simulink model "pll_d1"  (Simulink 7.4)
settings: Solver=ode45  StartTime=0.0  StopTime=6e-4  MaxStep=1/(10*50e6)  RelTol=1e-5  AbsTol=1e-6
PreLoadFcn:
  | load f_inv;   % 1/f filter kernel
undefined symbols (not defined in the file or in its folder): dfilt, One, sided
libraries: powerlib x11, dsparch4 x5, dspstat3 x5, simulink x4, simulink_extras x2, dspsnks4 x2, dspsrcs4 x1, dspbuff3 x1
settings Model: Creator=dbenson  LastModifiedBy=Dick  ExtModeTrigMode=oneshot  ExtModeArmWhenConnect=off
settings DataIOCC: LimitDataPoints=off  SaveOutput=off  SaveTime=off  SignalLoggingName=sigsOut
settings OptimizationCC: BooleanDataType=off  InitFltsAndDblsToZero=on
settings DebuggingCC: SaveWithParameterizedLinksMsg=none  SignalResolutionControl=TryResolveAllWithWarning  SolverPrmCheckMsg=none  MultiTaskDSMMsg=warning  MultiTaskCondExecSysMsg=none  StrictBusMsg=None
settings HardwareCC: TargetUnknown=on
settings RTWCC: RTWVerbose=off  IncludeERTFirstTime=on
settings CodeAppCC: GenerateComments=off  SimulinkBlockComments=off
settings GRTTargetCC: TargetFcnLib=ansi_tfl_tmw.mat

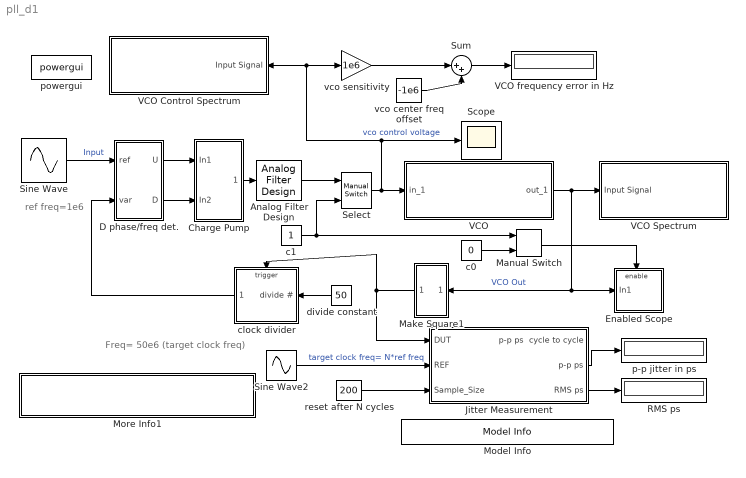
== system pll_d1 ==
  note: ref freq=1e6
  note: Freq= 50e6 (target clock freq)
  Analog Filter Design : dsparch4/Analog Filter Design  method=Butterworth  filttype=Lowpass  N=3  Wlo=2*pi*500e3  Whi=80  Rp=2  Rs=40
  Charge Pump : Subsystem  mask(RC Charge Pump){V=5}
      mask prompts: V "Output Voltage, V (Volts)"
  "D phase/freq det. " : Subsystem
  Enabled Scope : Subsystem  TreatAsAtomicUnit=on
  "Jitter Measurement " : Subsystem
  Make Square1 : Subsystem
      mask Type: Make Square
      mask Description:
      | For input +ve values output is 1
      | For input -ve values output is 0
      mask Display: plot(0,0,100,100,[90,70,70,50,50,30,30,10,10],[20,20,40,40,20,20,40,40,20],[90,87,84,80,76,73,70,67,63,60,57,53,50,47,44,40,36,33,30,27,23,20,17,13,10],[70,65,63,62,63,65,70,75,77,78,77,75,70,65,63,62,63,65,70,75,77,78,77,75,70])
  Manual Switch : simulink/Signal Routing/Manual Switch  SystemSampleTime=-1  sw=0  action=0  varsize=off
  Model Info : simulink/Model-Wide Utilities/Model Info  SystemSampleTime=-1  InitialBlockCM=none  BlockCM=none  Frame=on  DisplayStringWithTags=Copywrite 2005-2010 The MathWorks, Inc.  HorizontalTextAlignment=Center  LeftAlignmentValue=0.5  SourceBlockDiagram=pll_d1  TagMaxNumber=20
  More Info1 : Subsystem  AncestorBlock=rab_favorites/More Info1
      mask Display: disp(' x50  PLL model \n with time and \nfrequency domain measurements. ')
  RMS ps : Display
  Scope : Scope
      settings: TimeRange=0.0006  YMin=0  YMax=1.4  MaxDataPoints=50000  Decimation=500
  "Select " : simulink/Signal Routing/Manual Switch  SystemSampleTime=-1  sw=1  action=0  varsize=off
  Sine Wave : Sin  Amplitude=1  Bias=0  Frequency=2*pi*(1e6)  Phase=0  Samples=10  SampleTime=0  Offset=0
  Sine Wave2 : Sin  Amplitude=1  Bias=0  Frequency=2*pi*(50e6)  Phase=pi/2  Samples=10  SampleTime=0  Offset=0
  Sum : Sum  Inputs=|++  OutDataType=sfix(16)  OutScaling=2^0  SaturateOnIntegerOverflow=on  InputSameDT=on  OutDataTypeStr=Inherit: Same as first input
  VCO : Subsystem  mask{BW=100e3, Nrms=0 % 0.5, Ph=0, Kc=1e6, Fc=49e6, Ac=1}
      mask prompts: BW "Single Sided Noise BW (Hz)"; Nrms "Phase Noise Level (rms rad)"; Ph "Initial Phase (rad)"; Kc "Input Sensitivity (Hz/Volt)"; Fc "Oscillation freq (Hz)"; Ac "Output amplitude (Volt)"
      mask init:
      | pi2=2*pi;
      mask Display: disp('VCO with \n 1/F phase noise')
  VCO Control Spectrum : Subsystem  Description=Spectrum Analyzer  mask{BW=5e6}
      mask prompts: BW "Bandwidth"
      mask Display: fprintf('Baseband Spectrum Analyzer \n  BW=%7.2f MHz', BW/1e6)
  VCO Spectrum : Subsystem  Description=Spectrum Analyzer  mask{BW=5e6, Fc=1e6*50}
      mask prompts: BW "Bandwidth"; Fc "Center Freq"
      mask Display: fprintf('Spectrum Analyzer \n Fc=%7.2f MHz \n BW=%7.2f MHz',Fc/1e6,BW/1e6)
  VCO frequency error in Hz : Display
      settings: Decimation=401
  c0 : Constant  Value=0  OutDataType=sfix(16)  OutScaling=2^0
  c1 : Constant  OutDataType=sfix(16)  OutScaling=2^0
  clock divider : Subsystem  TreatAsAtomicUnit=on
  divide constant : Constant  Value=50  OutDataType=sfix(16)  OutScaling=2^0
  p-p jitter in ps : Display
  powergui : powerlib/powergui  SystemSampleTime=-1  SimulationMode=Continuous  SampleTime=0  frequency=60  SPID=off  DisableSnubberDevices=off  DisableRonSwitches=off  DisableVfSwitches=off  SwTol=0  Interpol=off  frequencyindice=0  echomessages=off  HookPort=off  DisplayEquations=off  FunctionMessages=off  EnableUseOfTLC=off  x0status=blocks  RestoreLinks=warning  Frange=[0:2:500]  Ylog=off  Xlog=on  ShowGrid=off  save=off  variable=ZData  ZoomFFT=on  StartTime=0.0  cycles=1  DisplayStyle=1  fundamental=60  FreqAxis=off  MaxFrequency=1000  frequencyindicesteady=1  RmsSteady=1  display=off  Ts=0  methode=off
  reset after N cycles : Constant  Value=200  VectorParams1D=off  OutDataType=sfix(16)  OutScaling=2^0
  vco center freq offset : Constant  Value=-1e6  OutDataType=sfix(16)  OutScaling=2^0
  vco sensitivity : Gain  Gain=1e6  ParameterDataType=sfix(16)  ParameterScaling=2^0  OutDataType=sfix(16)  OutScaling=2^0  SaturateOnIntegerOverflow=on  OutDataTypeStr=Inherit: Same as input  ParamDataTypeStr=Inherit: Same as input
  wires:
  Make Square1/1(Out1) -> clock divider/Trigger, "Jitter Measurement "/1(DUT)
  clock divider/1(" ") -> "D phase/freq det. "/2(var)
  Sine Wave/1 -> "D phase/freq det. "/1(ref)  "Input"
  Charge Pump/1(Out1) -> Analog Filter Design/1
  vco center freq offset/1 -> Sum/2
  Sum/1 -> VCO frequency error in Hz/1
  vco sensitivity/1 -> Sum/1
  VCO/1(out_1) -> VCO Spectrum/1(Input Signal), Make Square1/1(In1), Enabled Scope/1(In1)  "VCO Out"
  "Select "/1 -> Scope/1, vco sensitivity/1, VCO Control Spectrum/1(Input Signal), VCO/1(in_1)  "vco control voltage"
  c1/1 -> "Select "/2, Manual Switch/1
  "D phase/freq det. "/1(U) -> Charge Pump/1(In1)
  "D phase/freq det. "/2(D) -> Charge Pump/2(In2)
  Analog Filter Design/1 -> "Select "/1
  divide constant/1 -> clock divider/1("divide # ")
  Sine Wave2/1 -> "Jitter Measurement "/2(REF)  "target clock freq= N*ref freq"
  reset after N cycles/1 -> "Jitter Measurement "/3(Sample_Size)
  "Jitter Measurement "/2(p-p ps) -> p-p jitter in ps/1
  Manual Switch/1 -> Enabled Scope/Enable
  c0/1 -> Manual Switch/2
  "Jitter Measurement "/3(RMS ps) -> RMS ps/1

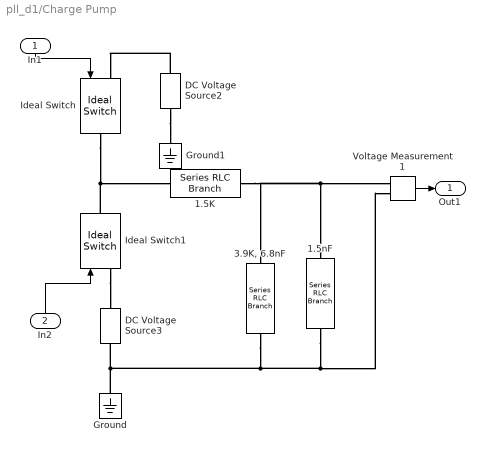
== system pll_d1/Charge Pump ==
  In1 : Inport  OutDataType=sfix(16)  OutScaling=2^0
  In2 : Inport  Port=2  OutDataType=sfix(16)  OutScaling=2^0
  1.5K : powerlib/Elements/Series RLC Branch  DialogController=POWERSYS.PowerSysDialog  PhysicalDomain=powersysdomain  SubClassName=unknown  LeftPortType=p1  RightPortType=p1  LConnTagsString=__new0  RConnTagsString=__new0  BranchType=R  Resistance=1500  Inductance=1e-3  SetiL0=off  InitialCurrent=0  Capacitance=1e-6  Setx0=off  InitialVoltage=0  Measurements=None
  1.5nF : powerlib/Elements/Series RLC Branch  DialogController=POWERSYS.PowerSysDialog  PhysicalDomain=powersysdomain  SubClassName=unknown  LeftPortType=p1  RightPortType=p1  LConnTagsString=__new0  RConnTagsString=__new0  BranchType=C  Resistance=3900  Inductance=1e-3  SetiL0=off  InitialCurrent=0  Capacitance=1.5e-9  Setx0=off  InitialVoltage=0  Measurements=None
  "3.9K, 6.8nF" : powerlib/Elements/Series RLC Branch  DialogController=POWERSYS.PowerSysDialog  PhysicalDomain=powersysdomain  SubClassName=unknown  LeftPortType=p1  RightPortType=p1  LConnTagsString=__new0  RConnTagsString=__new0  BranchType=RC  Resistance=3900  Inductance=1e-3  SetiL0=off  InitialCurrent=0  Capacitance=6.8e-9  Setx0=off  InitialVoltage=0  Measurements=None
  DC Voltage Source2 : powerlib/Electrical Sources/DC Voltage Source  DialogController=POWERSYS.PowerSysDialog  SystemSampleTime=-1  Amplitude=V  Measurements=None
  DC Voltage Source3 : powerlib/Electrical Sources/DC Voltage Source  DialogController=POWERSYS.PowerSysDialog  SystemSampleTime=-1  Amplitude=-V  Measurements=None
  Ground : powerlib/Elements/Ground  DialogController=POWERSYS.PowerSysDialog  PhysicalDomain=powersysdomain  SubClassName=unknown  LeftPortType=p1  RightPortType=p1  LConnTagsString=a
  Ground1 : powerlib/Elements/Ground  DialogController=POWERSYS.PowerSysDialog  PhysicalDomain=powersysdomain  SubClassName=unknown  LeftPortType=p1  RightPortType=p1  LConnTagsString=a
  Ideal Switch : powerlib/Power Electronics/Ideal Switch  DialogController=POWERSYS.PowerSysDialog  SystemSampleTime=-1  Ron=10  Lon=0  IC=0  Rs=inf  Cs=inf  Measurements=off
  Ideal Switch1 : powerlib/Power Electronics/Ideal Switch  DialogController=POWERSYS.PowerSysDialog  SystemSampleTime=-1  Ron=10  Lon=0  IC=0  Rs=inf  Cs=inf  Measurements=off
  Voltage Measurement1 : powerlib/Measurements/Voltage Measurement  DialogController=POWERSYS.PowerSysDialog  SystemSampleTime=-1  PhasorSimulation=off  OutputType=Complex  PSBequivalent=0
  Out1 : Outport  OutDataType=sfix(16)  OutScaling=2^0
  wires:
  In2/1 -> Ideal Switch1/1
  Voltage Measurement1/1 -> Out1/1
  In1/1 -> Ideal Switch/1
  connections:
  1.5nF/RConn1 -- "3.9K, 6.8nF"/RConn1 -- Ground/LConn1 -- DC Voltage Source3/LConn1 -- Voltage Measurement1/LConn2
  1.5K/RConn1 -- "3.9K, 6.8nF"/LConn1 -- Voltage Measurement1/LConn1 -- 1.5nF/LConn1
  Ideal Switch/RConn1 -- 1.5K/LConn1 -- Ideal Switch1/RConn1
  Ideal Switch1/LConn1 -- DC Voltage Source3/RConn1
  DC Voltage Source2/RConn1 -- Ideal Switch/LConn1
  DC Voltage Source2/LConn1 -- Ground1/LConn1

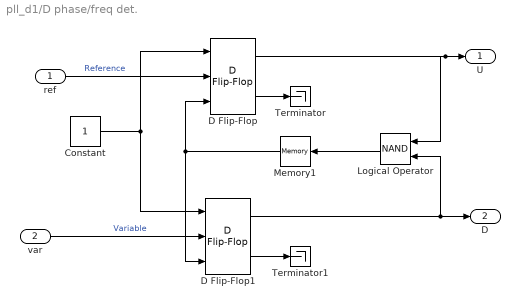
== system pll_d1/D phase/freq det.  ==
  ref : Inport  OutDataType=sfix(16)  OutScaling=2^0
  var : Inport  Port=2  OutDataType=sfix(16)  OutScaling=2^0
  Constant : Constant  OutDataType=sfix(16)  OutScaling=2^0
  D Flip-Flop : simulink_extras/Flip Flops/D Flip-Flop  SystemSampleTime=-1
  D Flip-Flop1 : simulink_extras/Flip Flops/D Flip-Flop  SystemSampleTime=-1
  Logical Operator : Logic  Operator=NAND
  Memory1 : Memory
  Terminator : Terminator
  Terminator1 : Terminator
  U : Outport  OutDataType=sfix(16)  OutScaling=2^0
  D : Outport  Port=2  OutDataType=sfix(16)  OutScaling=2^0
  wires:
  var/1 -> D Flip-Flop1/2  "Variable"
  D Flip-Flop/2 -> Terminator/1
  D Flip-Flop1/2 -> Terminator1/1
  ref/1 -> D Flip-Flop/2  "Reference"
  Constant/1 -> D Flip-Flop/1, D Flip-Flop1/1
  Memory1/1 -> D Flip-Flop/3, D Flip-Flop1/3
  D Flip-Flop/1 -> U/1, Logical Operator/1
  D Flip-Flop1/1 -> D/1, Logical Operator/2
  Logical Operator/1 -> Memory1/1

== system pll_d1/Enabled Scope ==
  In1 : Inport  OutDataType=sfix(16)  OutScaling=2^0
  Enable : EnablePort
  VCO Out (computationally expensive) : Scope
      settings: TimeRange=2e-008  YMin=-1  YMax=1  SaveName=ScopeData2  MaxDataPoints=500
  wires:
  In1/1 -> VCO Out (computationally expensive)/1

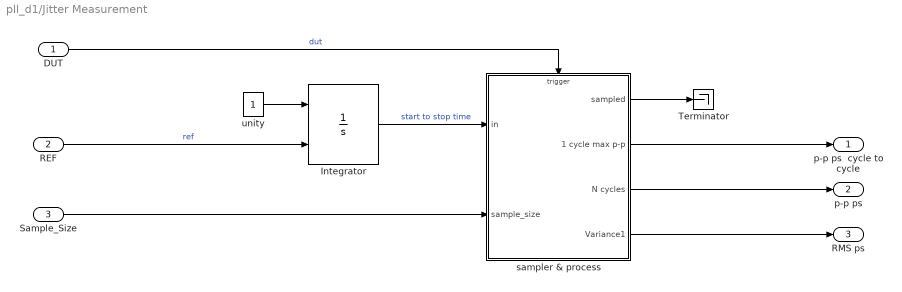
== system pll_d1/Jitter Measurement  ==
  DUT : Inport  OutDataType=sfix(16)  OutScaling=2^0
  REF : Inport  Port=2  OutDataType=sfix(16)  OutScaling=2^0
  Sample_Size : Inport  Port=3  OutDataType=sfix(16)  OutScaling=2^0
  Integrator : Integrator  ExternalReset=rising
  Terminator : Terminator
  sampler & process : Subsystem  TreatAsAtomicUnit=on
  unity : Constant  OutDataTypeMode=double  OutDataType=sfix(16)  OutScaling=2^0  OutDataTypeStr=double
  p-p ps  cycle to cycle : Outport  OutDataType=sfix(16)  OutScaling=2^0
  p-p ps : Outport  Port=2  OutDataType=sfix(16)  OutScaling=2^0
  RMS ps : Outport  Port=3  OutDataType=sfix(16)  OutScaling=2^0
  wires:
  DUT/1 -> sampler & process/Trigger  "dut"
  REF/1 -> Integrator/2  "ref"
  Integrator/1 -> sampler & process/1(in)  "start to stop time"
  Sample_Size/1 -> sampler & process/2(sample_size)
  sampler & process/3(N cycles) -> p-p ps/1
  sampler & process/4(Variance1) -> RMS ps/1
  unity/1 -> Integrator/1
  sampler & process/2(1 cycle max p-p) -> p-p ps  cycle to cycle/1
  sampler & process/1(sampled) -> Terminator/1

== system pll_d1/Make Square1 ==
  In1 : Inport  OutDataType=sfix(16)  OutScaling=2^0
  Constant : Constant  Value=0  OutDataType=sfix(16)  OutScaling=2^0
  Relational Operator : RelationalOperator  Operator=>  InputSameDT=on
  Out1 : Outport  OutDataType=sfix(16)  OutScaling=2^0
  wires:
  In1/1 -> Relational Operator/1
  Constant/1 -> Relational Operator/2
  Relational Operator/1 -> Out1/1

== system pll_d1/More Info1 ==
  note: This model multiplies the reference frequency of 1 MHz by
      | a factor of 50 using a phase lock loop.  It is virtually identical
      | to the pll_d0.mdl but includes spectrum analyzers to monitor the VCO
      | control voltage and VCO output signal. The VCO has a bandlimited phase
      | noise generator with a 1/f spectral shape, set by an FIR filter, to demonstrate
      | the effect of an imperfect VCO on spectral purity and time jitter.
      |
      | Points:
      | 1) Spectrum analyzers are made from the following blocks:
      |           a) continuous time low pass anti-alias filter
      |           b) sample and hold
      |           c) FFT (Spectrum Scope)
      |     A down converter (local oscillator and mixer) is used before
      |     the analyzer monitoring the VCO output to improve the frequency
      |     resolution of the analysis without going to excessively large
      |     record lengths.
      |
      | 2) When the simulation is run, and zero phase noise is specified for the VCO,
      |  the sidebands due to the 1 MHz reference along with other artifacts
      | around the VCO center frequency can be seen to diminish.
      |
      | 4)The  single period (20 ns) time history of the VCO output provides
      | a simple but effective display of the virtual absence of timeing jitter
      | when the loop has settled IF the phase noise of the VCO is set to zero.
      |
      | 5)  After the initial run, set the phase noise parameter of the VCO to
      | 0.5 rad rms.  Notice how the noise corrupts the spectral purity
      | of the VCO output. It is interesting to note that the noise also
      | causes the reference sidebands (+/- 1MHz around VCO freq) to
      | increase. This is typical behaviour of charge pump based phase-frequency
      | detector schemes. Be advised, enabling the phase noise will
      | slow down the simulation. Try the accelerator for improved performance.
  note: PLL with frequency domain measurements and imperfect VCO.

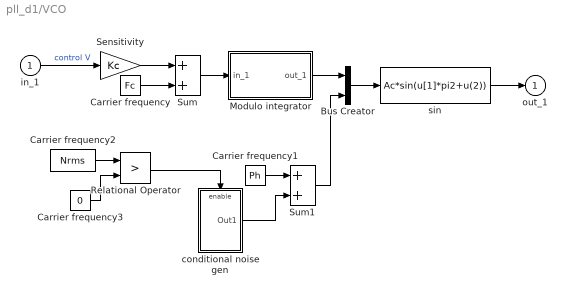
== system pll_d1/VCO ==
  in_1 : Inport  OutDataType=sfix(16)  OutScaling=2^0
  Bus Creator : BusCreator  Inputs=2
  Carrier frequency : Constant  Value=Fc  OutDataType=sfix(16)  OutScaling=2^0
  Carrier frequency1 : Constant  Value=Ph  OutDataType=sfix(16)  OutScaling=2^0
  Carrier frequency2 : Constant  Value=Nrms  OutDataType=sfix(16)  OutScaling=2^0
  Carrier frequency3 : Constant  Value=0  OutDataType=sfix(16)  OutScaling=2^0
  Modulo integrator : Subsystem  mask(Modulo integrator){modu=1, init=0}
      mask prompts: modu "Modulo bound:"; init "Initial state:"
      mask help: When the absolute value of the state exceeds the modulo bound, the state is reset to be the remainder of the state divided by the modulo bound.
      mask Help: This block calculate the integration of the input signal. The absolute value of this integrator will not exceed the specified module bound. The state value is reset to be the remainder of the state divided by the modulo bound. This block can only be used for scale value calculation. This block is a continuous-time integration block.
      mask Display: disp('Modulo\nintegrator')
  Relational Operator : RelationalOperator  Operator=>  InputSameDT=on
  Sensitivity : Gain  Gain=Kc  ParameterDataType=sfix(16)  ParameterScaling=2^0  OutDataType=sfix(16)  OutScaling=2^0  SaturateOnIntegerOverflow=on  OutDataTypeStr=Inherit: Same as input  ParamDataTypeStr=Inherit: Same as input
  Sum : Sum  OutDataType=sfix(16)  OutScaling=2^0  SaturateOnIntegerOverflow=on  InputSameDT=on  OutDataTypeStr=Inherit: Same as first input
  Sum1 : Sum  OutDataType=sfix(16)  OutScaling=2^0  SaturateOnIntegerOverflow=on  InputSameDT=on  OutDataTypeStr=Inherit: Same as first input
  conditional noise gen : Subsystem  TreatAsAtomicUnit=on
  sin : Fcn  Expr=Ac*sin(u[1]*pi2+u(2))
  out_1 : Outport  OutDataType=sfix(16)  OutScaling=2^0  InitialOutput=0
  wires:
  Modulo integrator/1(out_1) -> Bus Creator/1
  Bus Creator/1 -> sin/1
  Sum/1 -> Modulo integrator/1(in_1)
  sin/1 -> out_1/1
  Carrier frequency/1 -> Sum/2
  Sensitivity/1 -> Sum/1
  in_1/1 -> Sensitivity/1  "control V"
  Carrier frequency1/1 -> Sum1/1
  Sum1/1 -> Bus Creator/2
  conditional noise gen/1(Out1) -> Sum1/2
  Carrier frequency2/1 -> Relational Operator/1
  Relational Operator/1 -> conditional noise gen/Enable
  Carrier frequency3/1 -> Relational Operator/2

== system pll_d1/VCO Control Spectrum ==
  Input Signal : Inport  OutDataType=sfix(16)  OutScaling=2^0
  Spectrum Scope : dspsnks4/Spectrum Scope  DialogController=dspdialog.SpectrumScope  DialogControllerArgs=DataTag7  SystemSampleTime=-1  ScopeProperties=on  Domain=Frequency  HorizSpan=1  UseBuffer=on  BufferSize=256  Overlap=64  inpFftLenInherit=off  FFTlength=128  numAvg=2  DisplayProperties=off  AxisGrid=on  Memory=off  FrameNumber=on  AxisLegend=off  AxisZoom=off  OpenScopeAtSimStart=on  OpenScopeImmediately=off  FigPos=[496 197 384 215]  AxisProperties=off  XUnits=Hertz  XRange=One-sided ([0...Fs/2])  XDisplay=0  InheritXIncr=on  XIncr=1.0  XLabel=Samples  XLimit=Auto  YUnits=dBW  XMax=1  XMin=0  YLabel=dBW  LineProperties=off  wintypeSpecScope=Hann  RsSpecScope=50  betaSpecScope=5  winsampSpecScope=Periodic  XAxisParamsVer=6.8
      settings: YMin=-181.0721  YMax=-51.0721
  anti alias : dsparch4/Analog Filter Design  method=Elliptic  filttype=Lowpass  N=8  Wlo=BW*2*pi  Whi=80  Rp=0.11  Rs=100
  sampler : ZeroOrderHold  SampleTime=1/(2.56*BW)
  wires:
  Input Signal/1 -> anti alias/1
  anti alias/1 -> sampler/1
  sampler/1 -> Spectrum Scope/1

== system pll_d1/VCO Spectrum ==
  Input Signal : Inport  OutDataType=sfix(16)  OutScaling=2^0
  Sine Wave1 : Sin  Amplitude=2*sqrt(2)  Bias=0  Frequency=2*pi*(Fc-BW/2)  Phase=-pi/2  Samples=10  SampleTime=0  Offset=0
  Spectrum Scope : dspsnks4/Spectrum Scope  DialogController=dspdialog.SpectrumScope  DialogControllerArgs=DataTag8  SystemSampleTime=-1  ScopeProperties=on  Domain=Frequency  HorizSpan=1  UseBuffer=on  BufferSize=512  Overlap=256  inpFftLenInherit=off  FFTlength=128  numAvg=10  DisplayProperties=off  AxisGrid=on  Memory=off  FrameNumber=on  AxisLegend=off  AxisZoom=off  OpenScopeAtSimStart=on  OpenScopeImmediately=off  FigPos=[26 195 455 215]  AxisProperties=off  XUnits=Hertz  XRange=One-sided ([0...Fs/2])  XDisplay=0  InheritXIncr=on  XIncr=1.0  XLabel=Samples  XLimit=Auto  YUnits=dBW  XMax=1  XMin=0  YLabel=dBW  LineProperties=off  wintypeSpecScope=Hann  RsSpecScope=50  betaSpecScope=5  winsampSpecScope=Periodic  XAxisParamsVer=6.8
      settings: YMin=-100  YMax=0
  anti alias : dsparch4/Analog Filter Design  method=Elliptic  filttype=Lowpass  N=8  Wlo=BW*2*pi  Whi=80  Rp=0.11  Rs=100
  down convert : Product  OutDataType=sfix(16)  OutScaling=2^0  SaturateOnIntegerOverflow=on  InputSameDT=on  OutDataTypeStr=Inherit: Same as first input
  sampler : ZeroOrderHold  SampleTime=1/(2.56*BW)
  wires:
  Sine Wave1/1 -> down convert/1
  sampler/1 -> Spectrum Scope/1
  anti alias/1 -> sampler/1
  down convert/1 -> anti alias/1
  Input Signal/1 -> down convert/2

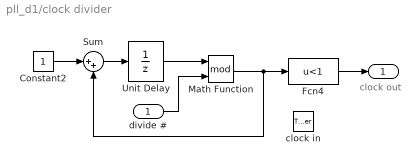
== system pll_d1/clock divider ==
  note: clock out
  "divide # " : Inport  OutDataType=sfix(16)  OutScaling=2^0
  clock in : TriggerPort
  Constant2 : Constant  OutDataType=sfix(16)  OutScaling=2^0
  Fcn4 : Fcn  Expr=u<1
  Math Function : Math  Operator=mod  OutDataType=sfix(16)  OutScaling=2^0  SaturateOnIntegerOverflow=on
  Sum : Sum  Inputs=|++  OutDataType=sfix(16)  OutScaling=2^0  SaturateOnIntegerOverflow=on  InputSameDT=on  OutDataTypeStr=Inherit: Same as first input
  Unit Delay : UnitDelay  SampleTime=-1
  " " : Outport  OutDataType=sfix(16)  OutScaling=2^0
  wires:
  "divide # "/1 -> Math Function/2
  Fcn4/1 -> " "/1
  Math Function/1 -> Fcn4/1, Sum/2
  Unit Delay/1 -> Math Function/1
  Constant2/1 -> Sum/1
  Sum/1 -> Unit Delay/1

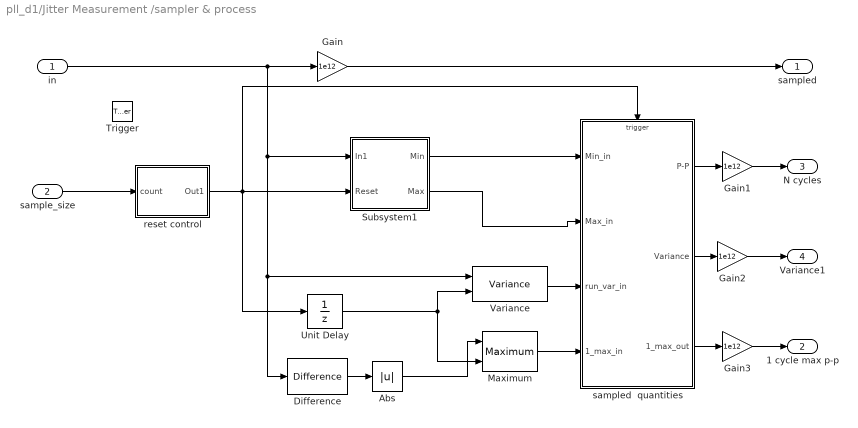
== system pll_d1/Jitter Measurement /sampler & process ==
  in : Inport  OutDataType=sfix(16)  OutScaling=2^0
  sample_size : Inport  Port=2  OutDataType=sfix(16)  OutScaling=2^0
  Trigger : TriggerPort
  Abs : Abs
  Difference : simulink/Discrete/Difference  SystemSampleTime=-1  ICPrevInput=0.0  OutMin=[]  OutMax=[]  OutDataType=sfix(16)  OutScaling=2^-10  DoSatur=off
  Gain{,1..3} (4 alike) : Gain  Gain=1e12  ParameterDataType=sfix(16)  ParameterScaling=2^0  OutDataType=sfix(16)  OutScaling=2^0
  Maximum : dspstat3/Maximum  DialogController=dspDDGCreate  DialogControllerArgs=DataTag0  fcn=Running  reset=Rising edge  indexBase=One  operateOver=Each column  Dimension=1  colComp=on  operation=maximum  roiEnable=off  roiType=Rectangles  roiPortion=Entire ROI  roiOutput=Individual statistics for each ROI  roiFlag=off  accumDataTypeStr=Inherit: Same as product output  accumLastDataTypeStr=Inherit: Same as product output  roundingMode=Floor  overflowMode=off
  Subsystem1 : Subsystem
  Unit Delay : UnitDelay  SampleTime=-1
  Variance : dspstat3/Variance  DialogController=dspDDGCreate  DialogControllerArgs=DataTag3  run=on  reset_popup=Rising edge  directionMode=Each column  dimension=1  treatSBRowAsCol=on  roiEnable=off  roiType=Rectangles  roiPortion=Entire ROI  roiOutput=Individual statistics for each ROI  roiFlag=off  roundingMode=Floor  overflowMode=off
  reset control : Subsystem
  sampled  quantities : Subsystem  TreatAsAtomicUnit=on
  sampled : Outport  OutDataType=sfix(16)  OutScaling=2^0
  1 cycle max p-p : Outport  Port=2  OutDataType=sfix(16)  OutScaling=2^0
  N cycles : Outport  Port=3  OutDataType=sfix(16)  OutScaling=2^0
  Variance1 : Outport  Port=4  OutDataType=sfix(16)  OutScaling=2^0
  wires:
  in/1 -> Gain/1, Variance/1, Difference/1, Subsystem1/1(In1)
  Difference/1 -> Abs/1
  Abs/1 -> Maximum/1
  sample_size/1 -> reset control/1(count)
  reset control/1(Out1) -> Unit Delay/1, sampled  quantities/Trigger, Subsystem1/2(Reset)
  sampled  quantities/1(P-P) -> Gain1/1
  Variance/1 -> sampled  quantities/3(run_var_in)
  sampled  quantities/2(Variance) -> Gain2/1
  Unit Delay/1 -> Variance/2, Maximum/2
  Maximum/1 -> sampled  quantities/4(1_max_in)
  sampled  quantities/3(1_max_out) -> Gain3/1
  Gain/1 -> sampled/1
  Gain1/1 -> N cycles/1
  Gain2/1 -> Variance1/1
  Gain3/1 -> 1 cycle max p-p/1
  Subsystem1/2(Max) -> sampled  quantities/2(Max_in)
  Subsystem1/1(Min) -> sampled  quantities/1(Min_in)

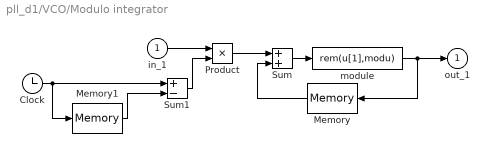
== system pll_d1/VCO/Modulo integrator ==
  in_1 : Inport  OutDataType=sfix(16)  OutScaling=2^0
  Clock : Clock
      settings: Decimation=10
  Memory : Memory  X0=init
  Memory1 : Memory
  Product : Product  OutDataType=sfix(16)  OutScaling=2^0  SaturateOnIntegerOverflow=on  InputSameDT=on  OutDataTypeStr=Inherit: Same as first input
  Sum : Sum  OutDataType=sfix(16)  OutScaling=2^0  SaturateOnIntegerOverflow=on  InputSameDT=on  OutDataTypeStr=Inherit: Same as first input
  Sum1 : Sum  Inputs=+-  OutDataType=sfix(16)  OutScaling=2^0  SaturateOnIntegerOverflow=on  InputSameDT=on  OutDataTypeStr=Inherit: Same as first input
  module : Fcn  Expr=rem(u[1],modu)
  out_1 : Outport  OutDataType=sfix(16)  OutScaling=2^0  InitialOutput=0
  wires:
  Memory1/1 -> Sum1/2
  Clock/1 -> Memory1/1, Sum1/1
  in_1/1 -> Product/1
  Sum1/1 -> Product/2
  Memory/1 -> Sum/2
  Product/1 -> Sum/1
  Sum/1 -> module/1
  module/1 -> out_1/1, Memory/1

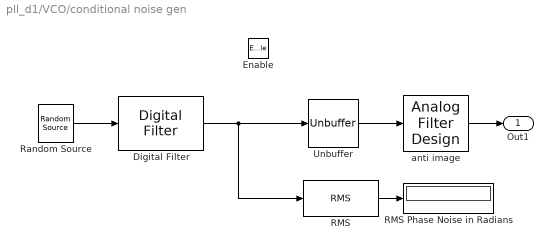
== system pll_d1/VCO/conditional noise gen ==
  Enable : EnablePort
  Digital Filter : dsparch4/Digital Filter  DialogController=dspdialog.DigitalFilter  DialogControllerArgs=DataTag4  TypePopup=FIR (all zeros)  IIRFiltStruct=Direct form II transposed  AllPoleFiltStruct=Direct form  FIRFiltStruct=Direct form  CoeffSource=Specify via dialog  NumCoeffs=f_inv  DenCoeffs=[1 0.1]  BiQuadCoeffs=[1 0.3 0.4 1 0.1 0.2]  LatticeCoeffs=[0.2 0.4]  denIgnore=on  FiltPerSampPopup=One filter per frame  IC=0  ICnum=0  ICden=0  roundingMode=Floor  overflowMode=off  ScaleValues=1  scaleValueFracLength=14  stageInFracLength=15  stageOutFracLength=15  FilterSource=Specify via dialog  dfiltObjectName=dfilt.dffir([1 2 1])
  RMS : dspstat3/RMS  DialogController=dspDDGCreate  DialogControllerArgs=DataTag5  run=off  reset_popup=None  directionMode=Each column  dimension=1  treatSBRowAsCol=on
  RMS Phase Noise in Radians : Display
  Random Source : dspsrcs4/Random Source  SrcType=Gaussian  NormMethod=Ziggurat  CltLength=12  MinVal=0  MaxVal=1  MeanVal=0  VarVal=(Nrms)^2+eps  RepMode=Not repeatable  rawSeed=1  IsInherit=off  SampMode=Discrete  SampTime=1/(2.56*BW)  SampFrame=512  DataType=Double  OutComplex=Real
  Unbuffer : dspbuff3/Unbuffer  ic=0
  anti image : dsparch4/Analog Filter Design  method=Elliptic  filttype=Lowpass  N=4  Wlo=BW*2*pi  Whi=80  Rp=2  Rs=100
  Out1 : Outport  OutDataType=sfix(16)  OutScaling=2^0
  wires:
  Random Source/1 -> Digital Filter/1
  Digital Filter/1 -> Unbuffer/1, RMS/1
  anti image/1 -> Out1/1
  Unbuffer/1 -> anti image/1
  RMS/1 -> RMS Phase Noise in Radians/1

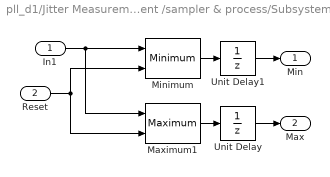
== system pll_d1/Jitter Measurement /sampler & process/Subsystem1 ==
  In1 : Inport  OutDataType=sfix(16)  OutScaling=2^0
  Reset : Inport  Port=2  OutDataType=sfix(16)  OutScaling=2^0
  Maximum1 : dspstat3/Maximum  DialogController=dspDDGCreate  DialogControllerArgs=DataTag1  fcn=Running  reset=Non-zero sample  indexBase=One  operateOver=Each column  Dimension=1  colComp=on  operation=maximum  roiEnable=off  roiType=Rectangles  roiPortion=Entire ROI  roiOutput=Individual statistics for each ROI  roiFlag=off  accumDataTypeStr=Inherit: Same as product output  accumLastDataTypeStr=Inherit: Same as product output  roundingMode=Floor  overflowMode=off
  Minimum : dspstat3/Minimum  DialogController=dspDDGCreate  DialogControllerArgs=DataTag2  fcn=Running  reset=Non-zero sample  indexBase=One  operateOver=Each column  Dimension=1  colComp=on  operation=minimum  roiEnable=off  roiType=Rectangles  roiPortion=Entire ROI  roiOutput=Individual statistics for each ROI  roiFlag=off  roundingMode=Floor  overflowMode=off
  Unit Delay : UnitDelay  SampleTime=-1
  Unit Delay1 : UnitDelay  SampleTime=-1
  Min : Outport  OutDataType=sfix(16)  OutScaling=2^0
  Max : Outport  Port=2  OutDataType=sfix(16)  OutScaling=2^0
  wires:
  Maximum1/1 -> Unit Delay/1
  Minimum/1 -> Unit Delay1/1
  Reset/1 -> Minimum/2, Maximum1/2
  In1/1 -> Minimum/1, Maximum1/1
  Unit Delay/1 -> Max/1
  Unit Delay1/1 -> Min/1

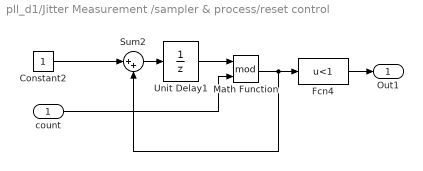
== system pll_d1/Jitter Measurement /sampler & process/reset control ==
  count : Inport  OutDataType=sfix(16)  OutScaling=2^0
  Constant2 : Constant  OutDataType=sfix(16)  OutScaling=2^0
  Fcn4 : Fcn  Expr=u<1
  Math Function : Math  Operator=mod  OutDataType=sfix(16)  OutScaling=2^0  SaturateOnIntegerOverflow=on
  Sum2 : Sum  Inputs=|++  OutDataType=sfix(16)  OutScaling=2^0  SaturateOnIntegerOverflow=on  InputSameDT=on  OutDataTypeStr=Inherit: Same as first input
  Unit Delay1 : UnitDelay  SampleTime=-1
  Out1 : Outport  OutDataType=sfix(16)  OutScaling=2^0
  wires:
  Math Function/1 -> Fcn4/1, Sum2/2
  Unit Delay1/1 -> Math Function/1
  Constant2/1 -> Sum2/1
  Sum2/1 -> Unit Delay1/1
  Fcn4/1 -> Out1/1
  count/1 -> Math Function/2

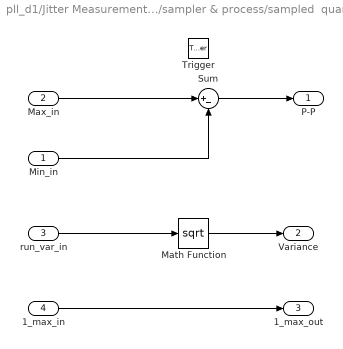
== system pll_d1/Jitter Measurement /sampler & process/sampled  quantities ==
  Min_in : Inport  OutDataType=sfix(16)  OutScaling=2^0
  Max_in : Inport  Port=2  OutDataType=sfix(16)  OutScaling=2^0
  run_var_in : Inport  Port=3  OutDataType=sfix(16)  OutScaling=2^0
  1_max_in : Inport  Port=4  OutDataType=sfix(16)  OutScaling=2^0
  Trigger : TriggerPort
  Math Function : Math  Operator=sqrt  OutDataType=sfix(16)  OutScaling=2^0  SaturateOnIntegerOverflow=on
  Sum : Sum  Inputs=|+-  OutDataType=sfix(16)  OutScaling=2^0  SaturateOnIntegerOverflow=on  InputSameDT=on  OutDataTypeStr=Inherit: Same as first input
  P-P : Outport  OutDataType=sfix(16)  OutScaling=2^0
  Variance : Outport  Port=2  OutDataType=sfix(16)  OutScaling=2^0
  1_max_out : Outport  Port=3  OutDataType=sfix(16)  OutScaling=2^0
  wires:
  Max_in/1 -> Sum/1
  Min_in/1 -> Sum/2
  Sum/1 -> P-P/1
  Math Function/1 -> Variance/1
  run_var_in/1 -> Math Function/1
  1_max_in/1 -> 1_max_out/1
